simulink model "CPG_component"  (R2021b)
settings: Solver=VariableStepAuto  StartTime=0.0  StopTime=5  RelTol=1e-3
values from neighbouring files (symbols this model uses):
  A = 2    [param.m]
  alpha = 0.856    [param.m]
  epsilon = 5    [param.m]
  f = 1/T    (= 0.8)    [param.m]
  init_state = rand(1, 8)*2 - 1    [param.m]
  k = 1000    [param.m]
  phi_vec = pi*[0; 0.5; 0; 0.5]    [param.m]
  tau = 0.5    [param.m]
settings Model: Creator=kaiget  LastModifiedBy=kaiget

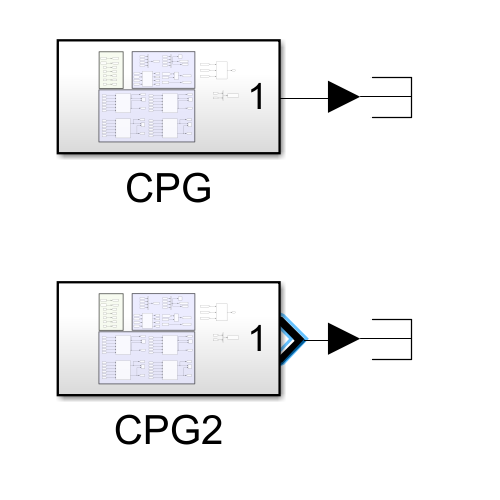
[thumbnail: Simulink's stored preview of the top-level diagram]
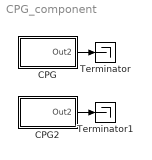
== system CPG_component ==
  CPG : Subsystem
  CPG2 : Subsystem
  Terminator : Terminator
  Terminator1 : Terminator
  wires:
  CPG/1(Out2) -> Terminator/1
  CPG2/1(Out2) -> Terminator1/1

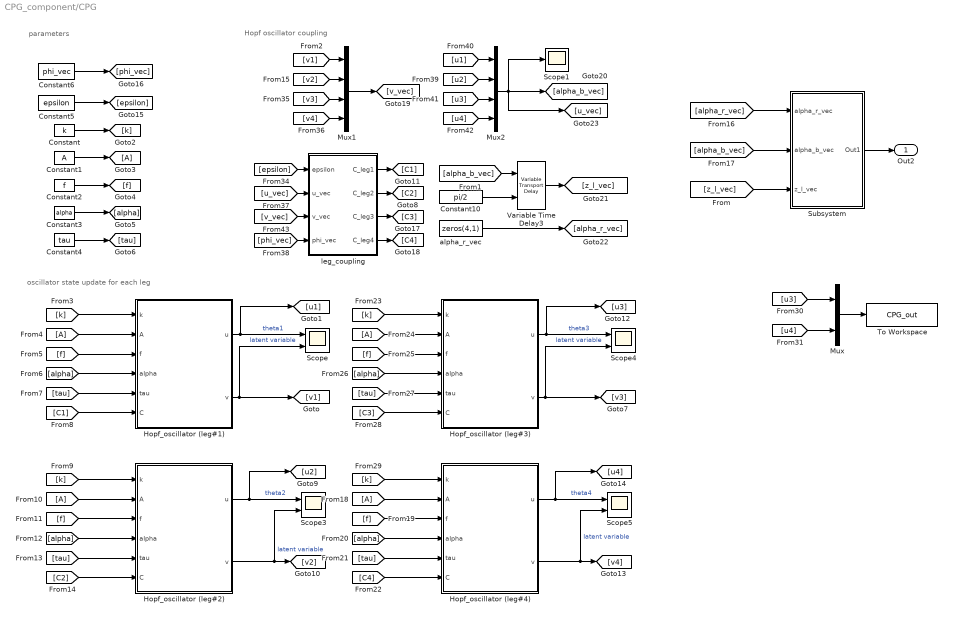
== system CPG_component/CPG ==
  note: oscillator state update for each leg
  note: Hopf oscillator coupling
  note: parameters
  Constant : Constant  Value=k
  Constant1 : Constant  Value=A
  Constant10 : Constant  Value=pi/2
  Constant2 : Constant  Value=f
  Constant3 : Constant  Value=alpha
  Constant4 : Constant  Value=tau
  Constant5 : Constant  Value=epsilon
  Constant6 : Constant  Value=phi_vec
  Hopf_oscillator (leg#1) : Subsystem
  Hopf_oscillator (leg#2) : Subsystem
  Hopf_oscillator (leg#3) : Subsystem
  Hopf_oscillator (leg#4) : Subsystem
  Mux : Mux  Inputs=2
  Mux1 : Mux
  Mux2 : Mux
  Scope{,3..5} (4 alike) : Scope  NumInputPorts=2
  Scope1 : Scope
  Subsystem : Subsystem
  To Workspace : ToWorkspace  VariableName=CPG_out  SaveFormat=Timeseries  SampleTime=0.01
  Variable Time Delay3 : VariableTransportDelay  MaximumDelay=10  MaximumPoints=4096  ZeroDelay=on
  alpha_r_vec : Constant  Value=zeros(4,1)
  leg_coupling : MATLAB Function  TreatAsAtomicUnit=on
  Out2 : Outport
  wires:
  [k] -> Hopf_oscillator (leg#4)/1(k)
  [tau] -> Hopf_oscillator (leg#3)/5(tau)
  [u4] -> Mux2/4
  [v2] -> Mux1/2
  Constant3/1 -> [alpha]
  [epsilon] -> leg_coupling/1(epsilon)
  [u3] -> Mux2/3
  [v_vec] -> leg_coupling/3(v_vec)
  [C2] -> Hopf_oscillator (leg#2)/6(C)
  leg_coupling/4(C_leg4) -> [C4]
  [f] -> Hopf_oscillator (leg#3)/3(f)
  Hopf_oscillator (leg#4)/1(u) -> [u4], Scope5/1  "theta4"
  Hopf_oscillator (leg#4)/2(v) -> [v4], Scope5/2  "latent variable"
  [k] -> Hopf_oscillator (leg#3)/1(k)
  leg_coupling/2(C_leg2) -> [C2]
  Constant2/1 -> [f]
  [u1] -> Mux2/1
  Hopf_oscillator (leg#3)/1(u) -> [u3], Scope4/1  "theta3"
  [A] -> Hopf_oscillator (leg#3)/2(A)
  leg_coupling/3(C_leg3) -> [C3]
  [u2] -> Mux2/2
  Hopf_oscillator (leg#1)/2(v) -> [v1], Scope/2  "latent variable"
  [alpha] -> Hopf_oscillator (leg#2)/4(alpha)
  Hopf_oscillator (leg#3)/2(v) -> [v3], Scope4/2  "latent variable"
  Constant4/1 -> [tau]
  [f] -> Hopf_oscillator (leg#2)/3(f)
  [tau] -> Hopf_oscillator (leg#4)/5(tau)
  [u_vec] -> leg_coupling/2(u_vec)
  [alpha] -> Hopf_oscillator (leg#3)/4(alpha)
  Constant1/1 -> [A]
  [A] -> Hopf_oscillator (leg#1)/2(A)
  [A] -> Hopf_oscillator (leg#2)/2(A)
  leg_coupling/1(C_leg1) -> [C1]
  Mux2/1 -> [u_vec], [alpha_b_vec], Scope1/1
  Hopf_oscillator (leg#2)/1(u) -> [u2], Scope3/1  "theta2"
  [v4] -> Mux1/4
  [f] -> Hopf_oscillator (leg#4)/3(f)
  [C4] -> Hopf_oscillator (leg#4)/6(C)
  [C3] -> Hopf_oscillator (leg#3)/6(C)
  [tau] -> Hopf_oscillator (leg#1)/5(tau)
  Constant5/1 -> [epsilon]
  [A] -> Hopf_oscillator (leg#4)/2(A)
  [k] -> Hopf_oscillator (leg#2)/1(k)
  [alpha] -> Hopf_oscillator (leg#4)/4(alpha)
  [v3] -> Mux1/3
  [k] -> Hopf_oscillator (leg#1)/1(k)
  [phi_vec] -> leg_coupling/4(phi_vec)
  [C1] -> Hopf_oscillator (leg#1)/6(C)
  [v1] -> Mux1/1
  Mux1/1 -> [v_vec]
  [tau] -> Hopf_oscillator (leg#2)/5(tau)
  [f] -> Hopf_oscillator (leg#1)/3(f)
  Constant/1 -> [k]
  Hopf_oscillator (leg#2)/2(v) -> [v2], Scope3/2  "latent variable"
  Hopf_oscillator (leg#1)/1(u) -> [u1], Scope/1  "theta1"
  [alpha] -> Hopf_oscillator (leg#1)/4(alpha)
  Constant6/1 -> [phi_vec]
  [alpha_b_vec] -> Variable Time Delay3/1
  Constant10/1 -> Variable Time Delay3/2
  Variable Time Delay3/1 -> [z_l_vec]
  alpha_r_vec/1 -> [alpha_r_vec]
  [alpha_r_vec] -> Subsystem/1(alpha_r_vec)
  [alpha_b_vec] -> Subsystem/2(alpha_b_vec)
  [z_l_vec] -> Subsystem/3(z_l_vec)
  Subsystem/1(Out1) -> Out2/1
  [u3] -> Mux/1
  [u4] -> Mux/2
  Mux/1 -> To Workspace/1

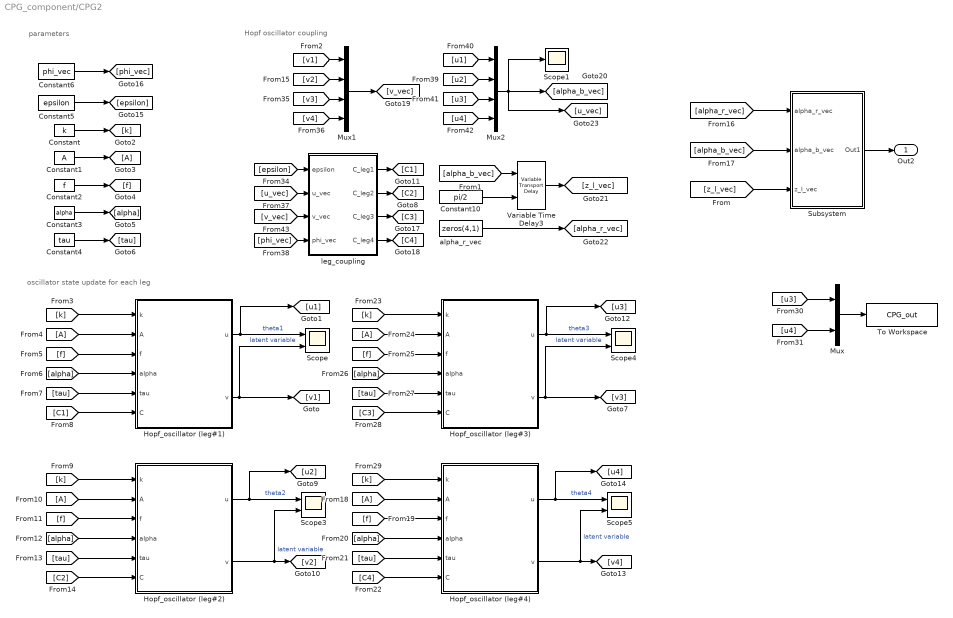
== system CPG_component/CPG2 ==
  note: oscillator state update for each leg
  note: Hopf oscillator coupling
  note: parameters
  Constant : Constant  Value=k
  Constant1 : Constant  Value=A
  Constant10 : Constant  Value=pi/2
  Constant2 : Constant  Value=f
  Constant3 : Constant  Value=alpha
  Constant4 : Constant  Value=tau
  Constant5 : Constant  Value=epsilon
  Constant6 : Constant  Value=phi_vec
  Hopf_oscillator (leg#1) : Subsystem
  Hopf_oscillator (leg#2) : Subsystem
  Hopf_oscillator (leg#3) : Subsystem
  Hopf_oscillator (leg#4) : Subsystem
  Mux : Mux  Inputs=2
  Mux1 : Mux
  Mux2 : Mux
  Scope{,3..5} (4 alike) : Scope  NumInputPorts=2
  Scope1 : Scope
  Subsystem : Subsystem
  To Workspace : ToWorkspace  VariableName=CPG_out  SaveFormat=Timeseries  SampleTime=0.01
  Variable Time Delay3 : VariableTransportDelay  MaximumDelay=10  MaximumPoints=4096  ZeroDelay=on
  alpha_r_vec : Constant  Value=zeros(4,1)
  leg_coupling : MATLAB Function  TreatAsAtomicUnit=on
  Out2 : Outport
  wires:
  [k] -> Hopf_oscillator (leg#4)/1(k)
  [tau] -> Hopf_oscillator (leg#3)/5(tau)
  [u4] -> Mux2/4
  [v2] -> Mux1/2
  Constant3/1 -> [alpha]
  [epsilon] -> leg_coupling/1(epsilon)
  [u3] -> Mux2/3
  [v_vec] -> leg_coupling/3(v_vec)
  [C2] -> Hopf_oscillator (leg#2)/6(C)
  leg_coupling/4(C_leg4) -> [C4]
  [f] -> Hopf_oscillator (leg#3)/3(f)
  Hopf_oscillator (leg#4)/1(u) -> [u4], Scope5/1  "theta4"
  Hopf_oscillator (leg#4)/2(v) -> [v4], Scope5/2  "latent variable"
  [k] -> Hopf_oscillator (leg#3)/1(k)
  leg_coupling/2(C_leg2) -> [C2]
  Constant2/1 -> [f]
  [u1] -> Mux2/1
  Hopf_oscillator (leg#3)/1(u) -> [u3], Scope4/1  "theta3"
  [A] -> Hopf_oscillator (leg#3)/2(A)
  leg_coupling/3(C_leg3) -> [C3]
  [u2] -> Mux2/2
  Hopf_oscillator (leg#1)/2(v) -> [v1], Scope/2  "latent variable"
  [alpha] -> Hopf_oscillator (leg#2)/4(alpha)
  Hopf_oscillator (leg#3)/2(v) -> [v3], Scope4/2  "latent variable"
  Constant4/1 -> [tau]
  [f] -> Hopf_oscillator (leg#2)/3(f)
  [tau] -> Hopf_oscillator (leg#4)/5(tau)
  [u_vec] -> leg_coupling/2(u_vec)
  [alpha] -> Hopf_oscillator (leg#3)/4(alpha)
  Constant1/1 -> [A]
  [A] -> Hopf_oscillator (leg#1)/2(A)
  [A] -> Hopf_oscillator (leg#2)/2(A)
  leg_coupling/1(C_leg1) -> [C1]
  Mux2/1 -> [u_vec], [alpha_b_vec], Scope1/1
  Hopf_oscillator (leg#2)/1(u) -> [u2], Scope3/1  "theta2"
  [v4] -> Mux1/4
  [f] -> Hopf_oscillator (leg#4)/3(f)
  [C4] -> Hopf_oscillator (leg#4)/6(C)
  [C3] -> Hopf_oscillator (leg#3)/6(C)
  [tau] -> Hopf_oscillator (leg#1)/5(tau)
  Constant5/1 -> [epsilon]
  [A] -> Hopf_oscillator (leg#4)/2(A)
  [k] -> Hopf_oscillator (leg#2)/1(k)
  [alpha] -> Hopf_oscillator (leg#4)/4(alpha)
  [v3] -> Mux1/3
  [k] -> Hopf_oscillator (leg#1)/1(k)
  [phi_vec] -> leg_coupling/4(phi_vec)
  [C1] -> Hopf_oscillator (leg#1)/6(C)
  [v1] -> Mux1/1
  Mux1/1 -> [v_vec]
  [tau] -> Hopf_oscillator (leg#2)/5(tau)
  [f] -> Hopf_oscillator (leg#1)/3(f)
  Constant/1 -> [k]
  Hopf_oscillator (leg#2)/2(v) -> [v2], Scope3/2  "latent variable"
  Hopf_oscillator (leg#1)/1(u) -> [u1], Scope/1  "theta1"
  [alpha] -> Hopf_oscillator (leg#1)/4(alpha)
  Constant6/1 -> [phi_vec]
  [alpha_b_vec] -> Variable Time Delay3/1
  Constant10/1 -> Variable Time Delay3/2
  Variable Time Delay3/1 -> [z_l_vec]
  alpha_r_vec/1 -> [alpha_r_vec]
  [alpha_r_vec] -> Subsystem/1(alpha_r_vec)
  [alpha_b_vec] -> Subsystem/2(alpha_b_vec)
  [z_l_vec] -> Subsystem/3(z_l_vec)
  Subsystem/1(Out1) -> Out2/1
  [u3] -> Mux/1
  [u4] -> Mux/2
  Mux/1 -> To Workspace/1

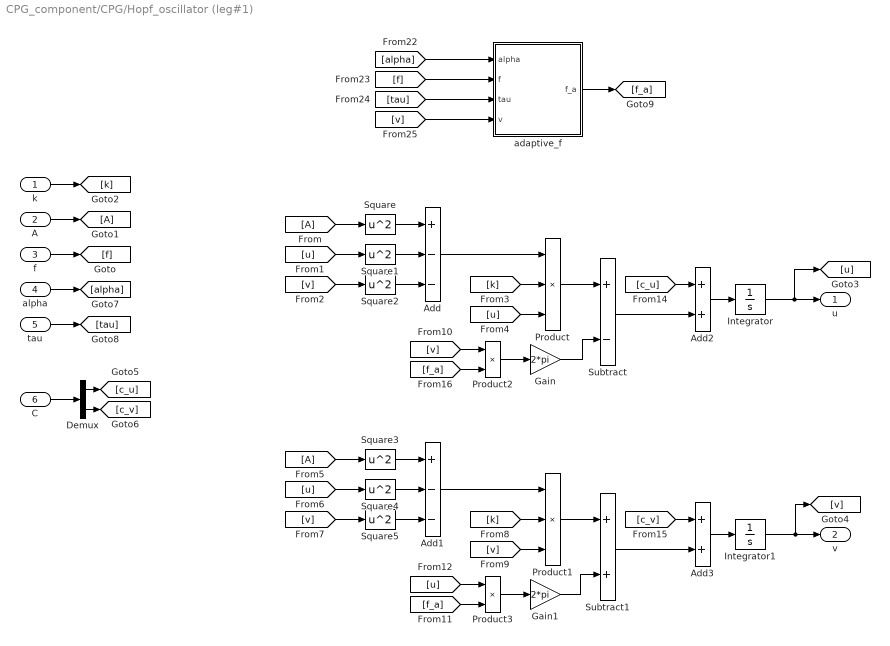
== system CPG_component/CPG/Hopf_oscillator (leg#1) ==
  k : Inport
  A : Inport  Port=2
  f : Inport  Port=3
  alpha : Inport  Port=4
  tau : Inport  Port=5
  C : Inport  Port=6
  Add : Sum  Inputs=+--
  Add1 : Sum  Inputs=+--
  Add2 : Sum
  Add3 : Sum
  Demux : Demux  Outputs=2
  Gain : Gain  Gain=2*pi
  Gain1 : Gain  Gain=2*pi
  Integrator : Integrator  InitialCondition=init_state(1)
  Integrator1 : Integrator  InitialCondition=init_state(2)
  Product : Product  Inputs=3
  Product1 : Product  Inputs=3
  Product2 : Product
  Product3 : Product
  Square{,1..5} (6 alike) : Math  Operator=square  SaturateOnIntegerOverflow=on
  Subtract : Sum  Inputs=+-
  Subtract1 : Sum
  adaptive_f : MATLAB Function  TreatAsAtomicUnit=on
  u : Outport
  v : Outport  Port=2
  wires:
  Integrator/1 -> [u], u/1
  f/1 -> [f]
  A/1 -> [A]
  k/1 -> [k]
  Integrator1/1 -> [v], v/1
  [A] -> Square/1
  [u] -> Square1/1
  [v] -> Square2/1
  Square2/1 -> Add/3
  Square1/1 -> Add/2
  Square/1 -> Add/1
  Add/1 -> Product/1
  [k] -> Product/2
  [u] -> Product/3
  Product/1 -> Subtract/1
  Square3/1 -> Add1/1
  Square4/1 -> Add1/2
  Square5/1 -> Add1/3
  [v] -> Product1/3
  Product1/1 -> Subtract1/1
  [v] -> Square5/1
  [A] -> Square3/1
  [u] -> Square4/1
  Add1/1 -> Product1/1
  [k] -> Product1/2
  [v] -> Product2/1
  [f_a] -> Product2/2
  Product2/1 -> Gain/1
  Gain/1 -> Subtract/2
  [u] -> Product3/1
  Product3/1 -> Gain1/1
  [f_a] -> Product3/2
  Gain1/1 -> Subtract1/2
  Subtract/1 -> Add2/2
  C/1 -> Demux/1
  Demux/1 -> [c_u]
  Demux/2 -> [c_v]
  [c_u] -> Add2/1
  Add2/1 -> Integrator/1
  Subtract1/1 -> Add3/2
  [c_v] -> Add3/1
  Add3/1 -> Integrator1/1
  alpha/1 -> [alpha]
  tau/1 -> [tau]
  [alpha] -> adaptive_f/1(alpha)
  [f] -> adaptive_f/2(f)
  [tau] -> adaptive_f/3(tau)
  [v] -> adaptive_f/4(v)
  adaptive_f/1(f_a) -> [f_a]

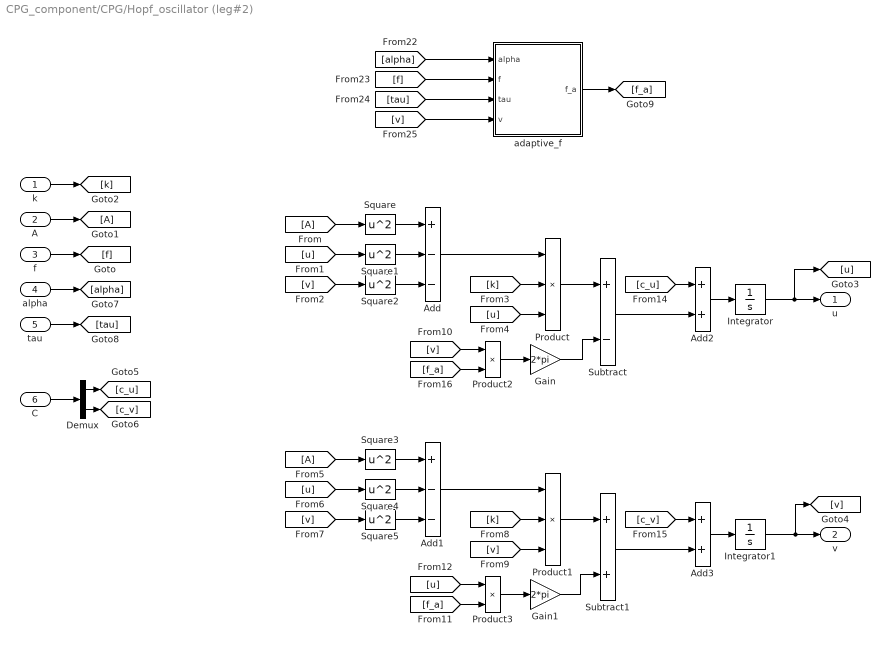
== system CPG_component/CPG/Hopf_oscillator (leg#2) ==
  k : Inport
  A : Inport  Port=2
  f : Inport  Port=3
  alpha : Inport  Port=4
  tau : Inport  Port=5
  C : Inport  Port=6
  Add : Sum  Inputs=+--
  Add1 : Sum  Inputs=+--
  Add2 : Sum
  Add3 : Sum
  Demux : Demux  Outputs=2
  Gain : Gain  Gain=2*pi
  Gain1 : Gain  Gain=2*pi
  Integrator : Integrator  InitialCondition=init_state(3)
  Integrator1 : Integrator  InitialCondition=init_state(4)
  Product : Product  Inputs=3
  Product1 : Product  Inputs=3
  Product2 : Product
  Product3 : Product
  Square{,1..5} (6 alike) : Math  Operator=square  SaturateOnIntegerOverflow=on
  Subtract : Sum  Inputs=+-
  Subtract1 : Sum
  adaptive_f : MATLAB Function  TreatAsAtomicUnit=on
  u : Outport
  v : Outport  Port=2
  wires:
  Integrator/1 -> [u], u/1
  f/1 -> [f]
  A/1 -> [A]
  k/1 -> [k]
  Integrator1/1 -> [v], v/1
  [A] -> Square/1
  [u] -> Square1/1
  [v] -> Square2/1
  Square2/1 -> Add/3
  Square1/1 -> Add/2
  Square/1 -> Add/1
  Add/1 -> Product/1
  [k] -> Product/2
  [u] -> Product/3
  Product/1 -> Subtract/1
  Square3/1 -> Add1/1
  Square4/1 -> Add1/2
  Square5/1 -> Add1/3
  [v] -> Product1/3
  Product1/1 -> Subtract1/1
  [v] -> Square5/1
  [A] -> Square3/1
  [u] -> Square4/1
  Add1/1 -> Product1/1
  [k] -> Product1/2
  [v] -> Product2/1
  [f_a] -> Product2/2
  Product2/1 -> Gain/1
  Gain/1 -> Subtract/2
  [u] -> Product3/1
  Product3/1 -> Gain1/1
  [f_a] -> Product3/2
  Gain1/1 -> Subtract1/2
  Subtract/1 -> Add2/2
  C/1 -> Demux/1
  Demux/1 -> [c_u]
  Demux/2 -> [c_v]
  [c_u] -> Add2/1
  Add2/1 -> Integrator/1
  Subtract1/1 -> Add3/2
  [c_v] -> Add3/1
  Add3/1 -> Integrator1/1
  alpha/1 -> [alpha]
  tau/1 -> [tau]
  [alpha] -> adaptive_f/1(alpha)
  [f] -> adaptive_f/2(f)
  [tau] -> adaptive_f/3(tau)
  [v] -> adaptive_f/4(v)
  adaptive_f/1(f_a) -> [f_a]

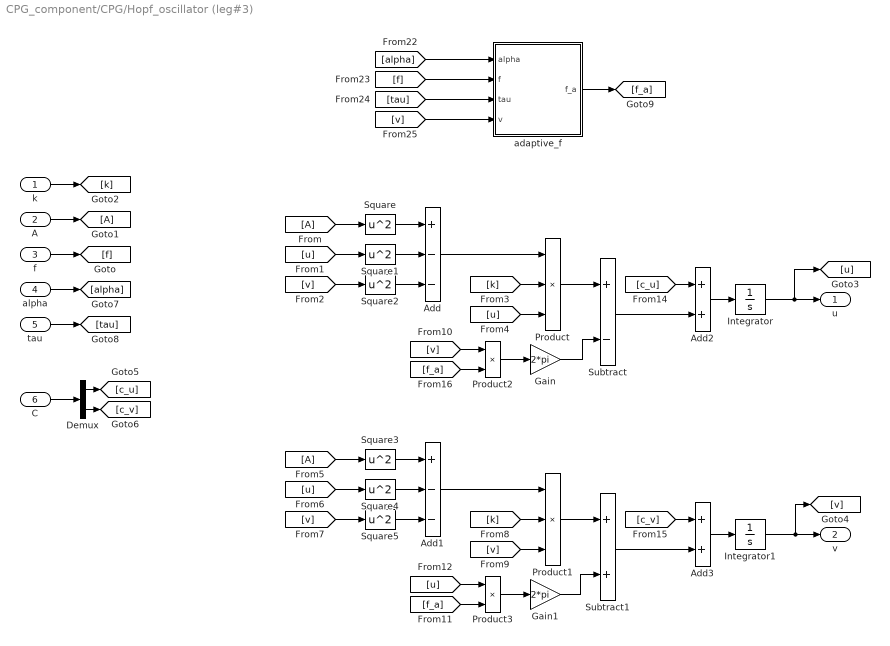
== system CPG_component/CPG/Hopf_oscillator (leg#3) ==
  k : Inport
  A : Inport  Port=2
  f : Inport  Port=3
  alpha : Inport  Port=4
  tau : Inport  Port=5
  C : Inport  Port=6
  Add : Sum  Inputs=+--
  Add1 : Sum  Inputs=+--
  Add2 : Sum
  Add3 : Sum
  Demux : Demux  Outputs=2
  Gain : Gain  Gain=2*pi
  Gain1 : Gain  Gain=2*pi
  Integrator : Integrator  InitialCondition=init_state(5)
  Integrator1 : Integrator  InitialCondition=init_state(6)
  Product : Product  Inputs=3
  Product1 : Product  Inputs=3
  Product2 : Product
  Product3 : Product
  Square{,1..5} (6 alike) : Math  Operator=square  SaturateOnIntegerOverflow=on
  Subtract : Sum  Inputs=+-
  Subtract1 : Sum
  adaptive_f : MATLAB Function  TreatAsAtomicUnit=on
  u : Outport
  v : Outport  Port=2
  wires:
  Integrator/1 -> [u], u/1
  f/1 -> [f]
  A/1 -> [A]
  k/1 -> [k]
  Integrator1/1 -> [v], v/1
  [A] -> Square/1
  [u] -> Square1/1
  [v] -> Square2/1
  Square2/1 -> Add/3
  Square1/1 -> Add/2
  Square/1 -> Add/1
  Add/1 -> Product/1
  [k] -> Product/2
  [u] -> Product/3
  Product/1 -> Subtract/1
  Square3/1 -> Add1/1
  Square4/1 -> Add1/2
  Square5/1 -> Add1/3
  [v] -> Product1/3
  Product1/1 -> Subtract1/1
  [v] -> Square5/1
  [A] -> Square3/1
  [u] -> Square4/1
  Add1/1 -> Product1/1
  [k] -> Product1/2
  [v] -> Product2/1
  [f_a] -> Product2/2
  Product2/1 -> Gain/1
  Gain/1 -> Subtract/2
  [u] -> Product3/1
  Product3/1 -> Gain1/1
  [f_a] -> Product3/2
  Gain1/1 -> Subtract1/2
  Subtract/1 -> Add2/2
  C/1 -> Demux/1
  Demux/1 -> [c_u]
  Demux/2 -> [c_v]
  [c_u] -> Add2/1
  Add2/1 -> Integrator/1
  Subtract1/1 -> Add3/2
  [c_v] -> Add3/1
  Add3/1 -> Integrator1/1
  alpha/1 -> [alpha]
  tau/1 -> [tau]
  [alpha] -> adaptive_f/1(alpha)
  [f] -> adaptive_f/2(f)
  [tau] -> adaptive_f/3(tau)
  [v] -> adaptive_f/4(v)
  adaptive_f/1(f_a) -> [f_a]

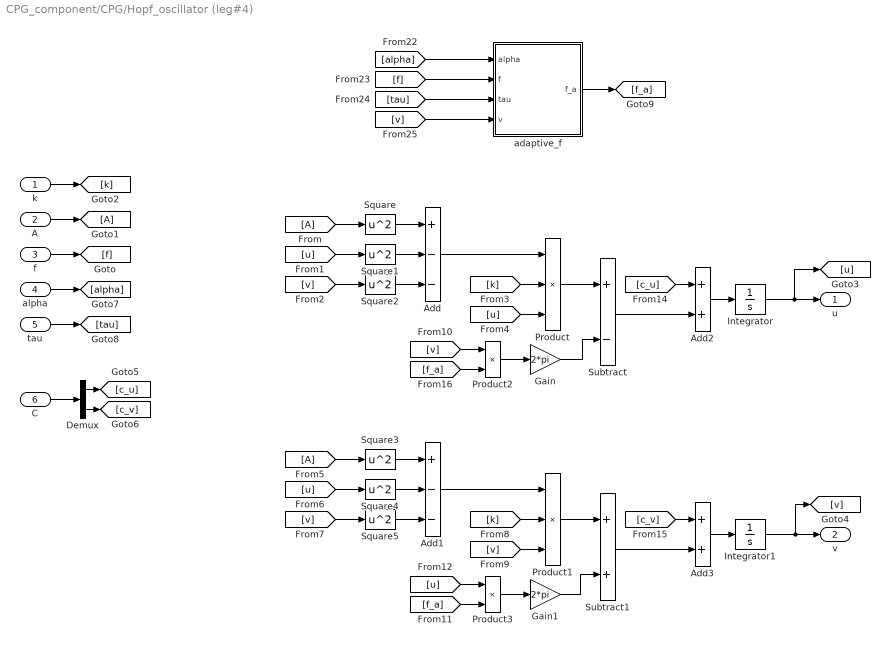
== system CPG_component/CPG/Hopf_oscillator (leg#4) ==
  k : Inport
  A : Inport  Port=2
  f : Inport  Port=3
  alpha : Inport  Port=4
  tau : Inport  Port=5
  C : Inport  Port=6
  Add : Sum  Inputs=+--
  Add1 : Sum  Inputs=+--
  Add2 : Sum
  Add3 : Sum
  Demux : Demux  Outputs=2
  Gain : Gain  Gain=2*pi
  Gain1 : Gain  Gain=2*pi
  Integrator : Integrator  InitialCondition=init_state(7)
  Integrator1 : Integrator  InitialCondition=init_state(8)
  Product : Product  Inputs=3
  Product1 : Product  Inputs=3
  Product2 : Product
  Product3 : Product
  Square{,1..5} (6 alike) : Math  Operator=square  SaturateOnIntegerOverflow=on
  Subtract : Sum  Inputs=+-
  Subtract1 : Sum
  adaptive_f : MATLAB Function  TreatAsAtomicUnit=on
  u : Outport
  v : Outport  Port=2
  wires:
  Integrator/1 -> [u], u/1
  f/1 -> [f]
  A/1 -> [A]
  k/1 -> [k]
  Integrator1/1 -> [v], v/1
  [A] -> Square/1
  [u] -> Square1/1
  [v] -> Square2/1
  Square2/1 -> Add/3
  Square1/1 -> Add/2
  Square/1 -> Add/1
  Add/1 -> Product/1
  [k] -> Product/2
  [u] -> Product/3
  Product/1 -> Subtract/1
  Square3/1 -> Add1/1
  Square4/1 -> Add1/2
  Square5/1 -> Add1/3
  [v] -> Product1/3
  Product1/1 -> Subtract1/1
  [v] -> Square5/1
  [A] -> Square3/1
  [u] -> Square4/1
  Add1/1 -> Product1/1
  [k] -> Product1/2
  [v] -> Product2/1
  [f_a] -> Product2/2
  Product2/1 -> Gain/1
  Gain/1 -> Subtract/2
  [u] -> Product3/1
  Product3/1 -> Gain1/1
  [f_a] -> Product3/2
  Gain1/1 -> Subtract1/2
  Subtract/1 -> Add2/2
  C/1 -> Demux/1
  Demux/1 -> [c_u]
  Demux/2 -> [c_v]
  [c_u] -> Add2/1
  Add2/1 -> Integrator/1
  Subtract1/1 -> Add3/2
  [c_v] -> Add3/1
  Add3/1 -> Integrator1/1
  alpha/1 -> [alpha]
  tau/1 -> [tau]
  [alpha] -> adaptive_f/1(alpha)
  [f] -> adaptive_f/2(f)
  [tau] -> adaptive_f/3(tau)
  [v] -> adaptive_f/4(v)
  adaptive_f/1(f_a) -> [f_a]

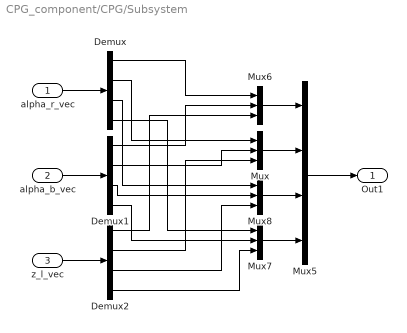
== system CPG_component/CPG/Subsystem ==
  alpha_r_vec : Inport
  alpha_b_vec : Inport  Port=2
  z_l_vec : Inport  Port=3
  Demux : Demux
  Demux1 : Demux
  Demux2 : Demux
  Mux{,6..8} (4 alike) : Mux  Inputs=3
  Mux5 : Mux
  Out1 : Outport
  wires:
  Mux6/1 -> Mux5/1
  Demux1/1 -> Mux6/2
  Demux/3 -> Mux8/1
  Demux2/1 -> Mux6/3
  alpha_b_vec/1 -> Demux1/1
  Demux/1 -> Mux6/1
  Demux2/4 -> Mux7/3
  Demux1/4 -> Mux7/2
  Demux/4 -> Mux7/1
  Mux5/1 -> Out1/1
  Demux2/3 -> Mux8/3
  Demux/2 -> Mux/1
  Mux8/1 -> Mux5/3
  Demux1/3 -> Mux8/2
  Demux1/2 -> Mux/2
  Mux7/1 -> Mux5/4
  Mux/1 -> Mux5/2
  Demux2/2 -> Mux/3
  z_l_vec/1 -> Demux2/1
  alpha_r_vec/1 -> Demux/1

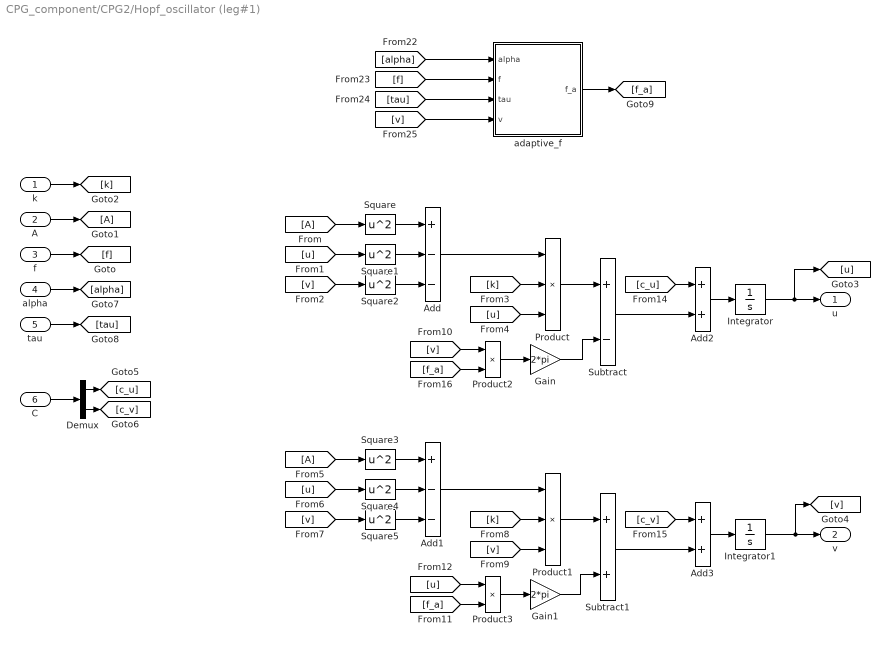
== system CPG_component/CPG2/Hopf_oscillator (leg#1) ==
  k : Inport
  A : Inport  Port=2
  f : Inport  Port=3
  alpha : Inport  Port=4
  tau : Inport  Port=5
  C : Inport  Port=6
  Add : Sum  Inputs=+--
  Add1 : Sum  Inputs=+--
  Add2 : Sum
  Add3 : Sum
  Demux : Demux  Outputs=2
  Gain : Gain  Gain=2*pi
  Gain1 : Gain  Gain=2*pi
  Integrator : Integrator  InitialCondition=init_state(1)
  Integrator1 : Integrator  InitialCondition=init_state(2)
  Product : Product  Inputs=3
  Product1 : Product  Inputs=3
  Product2 : Product
  Product3 : Product
  Square{,1..5} (6 alike) : Math  Operator=square  SaturateOnIntegerOverflow=on
  Subtract : Sum  Inputs=+-
  Subtract1 : Sum
  adaptive_f : MATLAB Function  TreatAsAtomicUnit=on
  u : Outport
  v : Outport  Port=2
  wires:
  Integrator/1 -> [u], u/1
  f/1 -> [f]
  A/1 -> [A]
  k/1 -> [k]
  Integrator1/1 -> [v], v/1
  [A] -> Square/1
  [u] -> Square1/1
  [v] -> Square2/1
  Square2/1 -> Add/3
  Square1/1 -> Add/2
  Square/1 -> Add/1
  Add/1 -> Product/1
  [k] -> Product/2
  [u] -> Product/3
  Product/1 -> Subtract/1
  Square3/1 -> Add1/1
  Square4/1 -> Add1/2
  Square5/1 -> Add1/3
  [v] -> Product1/3
  Product1/1 -> Subtract1/1
  [v] -> Square5/1
  [A] -> Square3/1
  [u] -> Square4/1
  Add1/1 -> Product1/1
  [k] -> Product1/2
  [v] -> Product2/1
  [f_a] -> Product2/2
  Product2/1 -> Gain/1
  Gain/1 -> Subtract/2
  [u] -> Product3/1
  Product3/1 -> Gain1/1
  [f_a] -> Product3/2
  Gain1/1 -> Subtract1/2
  Subtract/1 -> Add2/2
  C/1 -> Demux/1
  Demux/1 -> [c_u]
  Demux/2 -> [c_v]
  [c_u] -> Add2/1
  Add2/1 -> Integrator/1
  Subtract1/1 -> Add3/2
  [c_v] -> Add3/1
  Add3/1 -> Integrator1/1
  alpha/1 -> [alpha]
  tau/1 -> [tau]
  [alpha] -> adaptive_f/1(alpha)
  [f] -> adaptive_f/2(f)
  [tau] -> adaptive_f/3(tau)
  [v] -> adaptive_f/4(v)
  adaptive_f/1(f_a) -> [f_a]

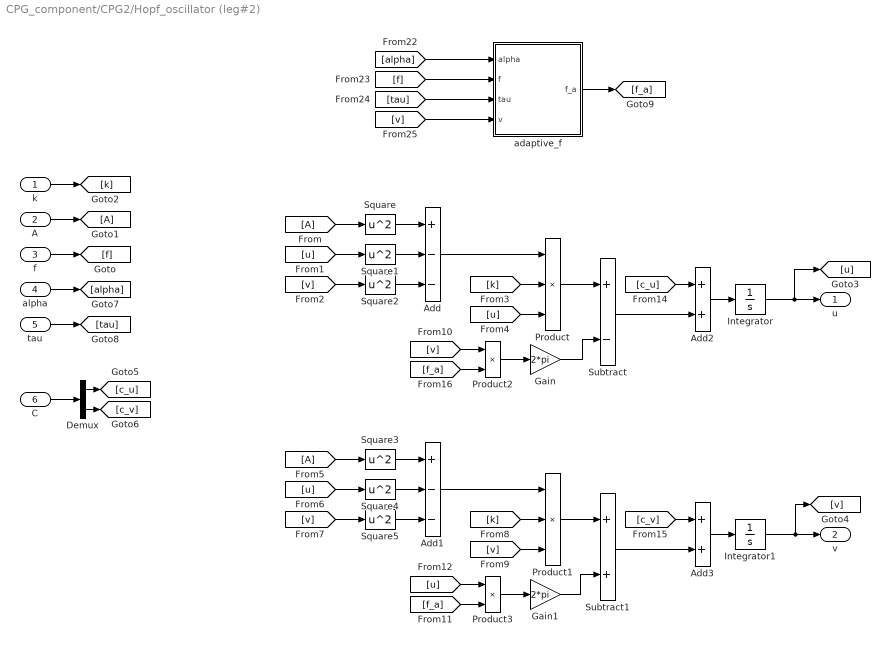
== system CPG_component/CPG2/Hopf_oscillator (leg#2) ==
  k : Inport
  A : Inport  Port=2
  f : Inport  Port=3
  alpha : Inport  Port=4
  tau : Inport  Port=5
  C : Inport  Port=6
  Add : Sum  Inputs=+--
  Add1 : Sum  Inputs=+--
  Add2 : Sum
  Add3 : Sum
  Demux : Demux  Outputs=2
  Gain : Gain  Gain=2*pi
  Gain1 : Gain  Gain=2*pi
  Integrator : Integrator  InitialCondition=init_state(3)
  Integrator1 : Integrator  InitialCondition=init_state(4)
  Product : Product  Inputs=3
  Product1 : Product  Inputs=3
  Product2 : Product
  Product3 : Product
  Square{,1..5} (6 alike) : Math  Operator=square  SaturateOnIntegerOverflow=on
  Subtract : Sum  Inputs=+-
  Subtract1 : Sum
  adaptive_f : MATLAB Function  TreatAsAtomicUnit=on
  u : Outport
  v : Outport  Port=2
  wires:
  Integrator/1 -> [u], u/1
  f/1 -> [f]
  A/1 -> [A]
  k/1 -> [k]
  Integrator1/1 -> [v], v/1
  [A] -> Square/1
  [u] -> Square1/1
  [v] -> Square2/1
  Square2/1 -> Add/3
  Square1/1 -> Add/2
  Square/1 -> Add/1
  Add/1 -> Product/1
  [k] -> Product/2
  [u] -> Product/3
  Product/1 -> Subtract/1
  Square3/1 -> Add1/1
  Square4/1 -> Add1/2
  Square5/1 -> Add1/3
  [v] -> Product1/3
  Product1/1 -> Subtract1/1
  [v] -> Square5/1
  [A] -> Square3/1
  [u] -> Square4/1
  Add1/1 -> Product1/1
  [k] -> Product1/2
  [v] -> Product2/1
  [f_a] -> Product2/2
  Product2/1 -> Gain/1
  Gain/1 -> Subtract/2
  [u] -> Product3/1
  Product3/1 -> Gain1/1
  [f_a] -> Product3/2
  Gain1/1 -> Subtract1/2
  Subtract/1 -> Add2/2
  C/1 -> Demux/1
  Demux/1 -> [c_u]
  Demux/2 -> [c_v]
  [c_u] -> Add2/1
  Add2/1 -> Integrator/1
  Subtract1/1 -> Add3/2
  [c_v] -> Add3/1
  Add3/1 -> Integrator1/1
  alpha/1 -> [alpha]
  tau/1 -> [tau]
  [alpha] -> adaptive_f/1(alpha)
  [f] -> adaptive_f/2(f)
  [tau] -> adaptive_f/3(tau)
  [v] -> adaptive_f/4(v)
  adaptive_f/1(f_a) -> [f_a]

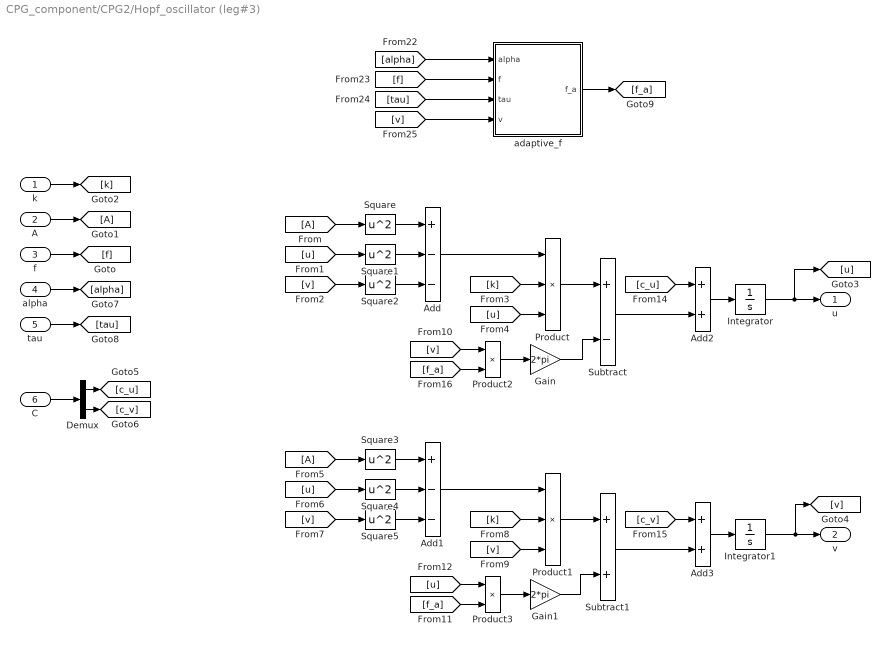
== system CPG_component/CPG2/Hopf_oscillator (leg#3) ==
  k : Inport
  A : Inport  Port=2
  f : Inport  Port=3
  alpha : Inport  Port=4
  tau : Inport  Port=5
  C : Inport  Port=6
  Add : Sum  Inputs=+--
  Add1 : Sum  Inputs=+--
  Add2 : Sum
  Add3 : Sum
  Demux : Demux  Outputs=2
  Gain : Gain  Gain=2*pi
  Gain1 : Gain  Gain=2*pi
  Integrator : Integrator  InitialCondition=init_state(5)
  Integrator1 : Integrator  InitialCondition=init_state(6)
  Product : Product  Inputs=3
  Product1 : Product  Inputs=3
  Product2 : Product
  Product3 : Product
  Square{,1..5} (6 alike) : Math  Operator=square  SaturateOnIntegerOverflow=on
  Subtract : Sum  Inputs=+-
  Subtract1 : Sum
  adaptive_f : MATLAB Function  TreatAsAtomicUnit=on
  u : Outport
  v : Outport  Port=2
  wires:
  Integrator/1 -> [u], u/1
  f/1 -> [f]
  A/1 -> [A]
  k/1 -> [k]
  Integrator1/1 -> [v], v/1
  [A] -> Square/1
  [u] -> Square1/1
  [v] -> Square2/1
  Square2/1 -> Add/3
  Square1/1 -> Add/2
  Square/1 -> Add/1
  Add/1 -> Product/1
  [k] -> Product/2
  [u] -> Product/3
  Product/1 -> Subtract/1
  Square3/1 -> Add1/1
  Square4/1 -> Add1/2
  Square5/1 -> Add1/3
  [v] -> Product1/3
  Product1/1 -> Subtract1/1
  [v] -> Square5/1
  [A] -> Square3/1
  [u] -> Square4/1
  Add1/1 -> Product1/1
  [k] -> Product1/2
  [v] -> Product2/1
  [f_a] -> Product2/2
  Product2/1 -> Gain/1
  Gain/1 -> Subtract/2
  [u] -> Product3/1
  Product3/1 -> Gain1/1
  [f_a] -> Product3/2
  Gain1/1 -> Subtract1/2
  Subtract/1 -> Add2/2
  C/1 -> Demux/1
  Demux/1 -> [c_u]
  Demux/2 -> [c_v]
  [c_u] -> Add2/1
  Add2/1 -> Integrator/1
  Subtract1/1 -> Add3/2
  [c_v] -> Add3/1
  Add3/1 -> Integrator1/1
  alpha/1 -> [alpha]
  tau/1 -> [tau]
  [alpha] -> adaptive_f/1(alpha)
  [f] -> adaptive_f/2(f)
  [tau] -> adaptive_f/3(tau)
  [v] -> adaptive_f/4(v)
  adaptive_f/1(f_a) -> [f_a]

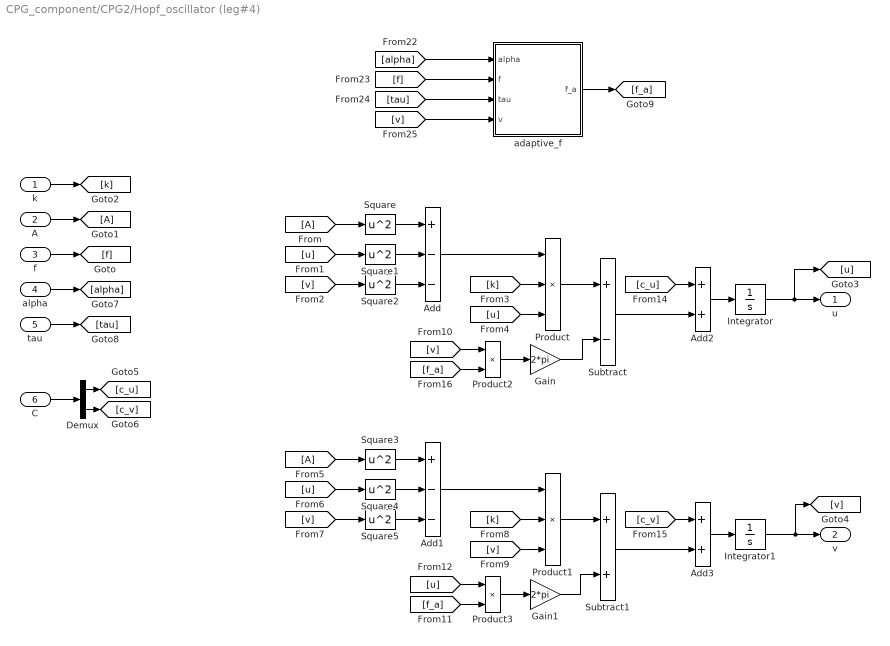
== system CPG_component/CPG2/Hopf_oscillator (leg#4) ==
  k : Inport
  A : Inport  Port=2
  f : Inport  Port=3
  alpha : Inport  Port=4
  tau : Inport  Port=5
  C : Inport  Port=6
  Add : Sum  Inputs=+--
  Add1 : Sum  Inputs=+--
  Add2 : Sum
  Add3 : Sum
  Demux : Demux  Outputs=2
  Gain : Gain  Gain=2*pi
  Gain1 : Gain  Gain=2*pi
  Integrator : Integrator  InitialCondition=init_state(7)
  Integrator1 : Integrator  InitialCondition=init_state(8)
  Product : Product  Inputs=3
  Product1 : Product  Inputs=3
  Product2 : Product
  Product3 : Product
  Square{,1..5} (6 alike) : Math  Operator=square  SaturateOnIntegerOverflow=on
  Subtract : Sum  Inputs=+-
  Subtract1 : Sum
  adaptive_f : MATLAB Function  TreatAsAtomicUnit=on
  u : Outport
  v : Outport  Port=2
  wires:
  Integrator/1 -> [u], u/1
  f/1 -> [f]
  A/1 -> [A]
  k/1 -> [k]
  Integrator1/1 -> [v], v/1
  [A] -> Square/1
  [u] -> Square1/1
  [v] -> Square2/1
  Square2/1 -> Add/3
  Square1/1 -> Add/2
  Square/1 -> Add/1
  Add/1 -> Product/1
  [k] -> Product/2
  [u] -> Product/3
  Product/1 -> Subtract/1
  Square3/1 -> Add1/1
  Square4/1 -> Add1/2
  Square5/1 -> Add1/3
  [v] -> Product1/3
  Product1/1 -> Subtract1/1
  [v] -> Square5/1
  [A] -> Square3/1
  [u] -> Square4/1
  Add1/1 -> Product1/1
  [k] -> Product1/2
  [v] -> Product2/1
  [f_a] -> Product2/2
  Product2/1 -> Gain/1
  Gain/1 -> Subtract/2
  [u] -> Product3/1
  Product3/1 -> Gain1/1
  [f_a] -> Product3/2
  Gain1/1 -> Subtract1/2
  Subtract/1 -> Add2/2
  C/1 -> Demux/1
  Demux/1 -> [c_u]
  Demux/2 -> [c_v]
  [c_u] -> Add2/1
  Add2/1 -> Integrator/1
  Subtract1/1 -> Add3/2
  [c_v] -> Add3/1
  Add3/1 -> Integrator1/1
  alpha/1 -> [alpha]
  tau/1 -> [tau]
  [alpha] -> adaptive_f/1(alpha)
  [f] -> adaptive_f/2(f)
  [tau] -> adaptive_f/3(tau)
  [v] -> adaptive_f/4(v)
  adaptive_f/1(f_a) -> [f_a]

== system CPG_component/CPG2/Subsystem ==
  alpha_r_vec : Inport
  alpha_b_vec : Inport  Port=2
  z_l_vec : Inport  Port=3
  Demux : Demux
  Demux1 : Demux
  Demux2 : Demux
  Mux{,6..8} (4 alike) : Mux  Inputs=3
  Mux5 : Mux
  Out1 : Outport
  wires:
  Mux6/1 -> Mux5/1
  Demux1/1 -> Mux6/2
  Demux/3 -> Mux8/1
  Demux2/1 -> Mux6/3
  alpha_b_vec/1 -> Demux1/1
  Demux/1 -> Mux6/1
  Demux2/4 -> Mux7/3
  Demux1/4 -> Mux7/2
  Demux/4 -> Mux7/1
  Mux5/1 -> Out1/1
  Demux2/3 -> Mux8/3
  Demux/2 -> Mux/1
  Mux8/1 -> Mux5/3
  Demux1/3 -> Mux8/2
  Demux1/2 -> Mux/2
  Mux7/1 -> Mux5/4
  Mux/1 -> Mux5/2
  Demux2/2 -> Mux/3
  z_l_vec/1 -> Demux2/1
  alpha_r_vec/1 -> Demux/1

== matlab function CPG_component/CPG/leg_coupling ==
  data: epsilon input; u_vec input; C_leg1 output size=2; v_vec input; phi_vec input; C_leg2 output size=2; C_leg3 output size=2; C_leg4 output size=2
% epsilon: 1X1
% u_vec: 4X1
% v_vec: 4X1
% phi_vec: 4X1
% C_leg1-4 : 2X1
function [C_leg1, C_leg2, C_leg3, C_leg4] = fcn(epsilon, u_vec, v_vec, phi_vec)
    C1 = 0;
    % first leg
    C21 = epsilon*(-u_vec(4)*sin(phi_vec(4)) + v_vec(4)*cos(phi_vec(4)) - ...
                   -u_vec(1)*sin(phi_vec(1)) + v_vec(2)*cos(phi_vec(1)));
    C22 = epsilon*(-u_vec(1)*sin(phi_vec(1)) + v_vec(1)*cos(phi_vec(1)) - ...
                   -u_vec(2)*sin(phi_vec(2)) + v_vec(3)*cos(phi_vec(2)));
    C23 = epsilon*(-u_vec(2)*sin(phi_vec(2)) + v_vec(2)*cos(phi_vec(2)) - ...
                   -u_vec(3)*sin(phi_vec(3)) + v_vec(4)*cos(phi_vec(3)));
    C24 = epsilon*(-u_vec(3)*sin(phi_vec(3)) + v_vec(3)*cos(phi_vec(3)) - ...
                   -u_vec(4)*sin(phi_vec(4)) + v_vec(1)*cos(phi_vec(4)));
    
    C_leg1 = [C1; C21];
    C_leg2 = [C1; C22];
    C_leg3 = [C1; C23];
    C_leg4 = [C1; C24];

== matlab function CPG_component/CPG2/Hopf_oscillator (leg#1)/adaptive_f ==
  data: alpha input; f_a output; f input; tau input; v input
 % calculate the adaptive frequency f through (4) in 
 % 'Design and Locomotion Control of a Biomimetic Underwater Vehicle ... '
function f_a = adaptive_f(alpha, f, tau, v)
    f1 = f/2/alpha;
    f2 = (2*alpha - 1)*f/(2*alpha*(1 - alpha)*(1 + exp(-tau*v)));
    f_a = f1 + f2;

== matlab function CPG_component/CPG2/Hopf_oscillator (leg#2)/adaptive_f ==
  data: alpha input; f_a output; f input; tau input; v input
 % calculate the adaptive frequency f through (4) in 
 % 'Design and Locomotion Control of a Biomimetic Underwater Vehicle ... '
function f_a = adaptive_f(alpha, f, tau, v)
    f1 = f/2/alpha;
    f2 = (2*alpha - 1)*f/(2*alpha*(1 - alpha)*(1 + exp(-tau*v)));
    f_a = f1 + f2;

== matlab function CPG_component/CPG2/Hopf_oscillator (leg#3)/adaptive_f ==
  data: alpha input; f_a output; f input; tau input; v input
 % calculate the adaptive frequency f through (4) in 
 % 'Design and Locomotion Control of a Biomimetic Underwater Vehicle ... '
function f_a = adaptive_f(alpha, f, tau, v)
    f1 = f/2/alpha;
    f2 = (2*alpha - 1)*f/(2*alpha*(1 - alpha)*(1 + exp(-tau*v)));
    f_a = f1 + f2;

== matlab function CPG_component/CPG2/Hopf_oscillator (leg#4)/adaptive_f ==
  data: alpha input; f_a output; f input; tau input; v input
 % calculate the adaptive frequency f through (4) in 
 % 'Design and Locomotion Control of a Biomimetic Underwater Vehicle ... '
function f_a = adaptive_f(alpha, f, tau, v)
    f1 = f/2/alpha;
    f2 = (2*alpha - 1)*f/(2*alpha*(1 - alpha)*(1 + exp(-tau*v)));
    f_a = f1 + f2;

== matlab function CPG_component/CPG2/leg_coupling ==
  data: epsilon input; u_vec input; C_leg1 output size=2; v_vec input; phi_vec input; C_leg2 output size=2; C_leg3 output size=2; C_leg4 output size=2
% epsilon: 1X1
% u_vec: 4X1
% v_vec: 4X1
% phi_vec: 4X1
% C_leg1-4 : 2X1
function [C_leg1, C_leg2, C_leg3, C_leg4] = fcn(epsilon, u_vec, v_vec, phi_vec)
    C1 = 0;
    % first leg
    C21 = 0;
    C22 = epsilon*(u_vec(1)*sin(phi_vec(2)) + v_vec(1)*cos(phi_vec(2)));
    C23 = epsilon*(u_vec(1)*sin(phi_vec(3)) + v_vec(1)*cos(phi_vec(3)));
    C24 = epsilon*(u_vec(1)*sin(phi_vec(4)) + v_vec(1)*cos(phi_vec(4)));
    
    C_leg1 = [C1; C21];
    C_leg2 = [C1; C22];
    C_leg3 = [C1; C23];
    C_leg4 = [C1; C24];

== matlab function CPG_component/CPG/Hopf_oscillator (leg#1)/adaptive_f ==
  data: alpha input; f_a output; f input; tau input; v input
 % calculate the adaptive frequency f through (4) in 
 % 'Design and Locomotion Control of a Biomimetic Underwater Vehicle ... '
function f_a = adaptive_f(alpha, f, tau, v)
    f1 = f/2/alpha;
    f2 = (2*alpha - 1)*f/(2*alpha*(1 - alpha)*(1 + exp(-tau*v)));
    f_a = f1 + f2;

== matlab function CPG_component/CPG/Hopf_oscillator (leg#2)/adaptive_f ==
  data: alpha input; f_a output; f input; tau input; v input
 % calculate the adaptive frequency f through (4) in 
 % 'Design and Locomotion Control of a Biomimetic Underwater Vehicle ... '
function f_a = adaptive_f(alpha, f, tau, v)
    f1 = f/2/alpha;
    f2 = (2*alpha - 1)*f/(2*alpha*(1 - alpha)*(1 + exp(-tau*v)));
    f_a = f1 + f2;

== matlab function CPG_component/CPG/Hopf_oscillator (leg#3)/adaptive_f ==
  data: alpha input; f_a output; f input; tau input; v input
 % calculate the adaptive frequency f through (4) in 
 % 'Design and Locomotion Control of a Biomimetic Underwater Vehicle ... '
function f_a = adaptive_f(alpha, f, tau, v)
    f1 = f/2/alpha;
    f2 = (2*alpha - 1)*f/(2*alpha*(1 - alpha)*(1 + exp(-tau*v)));
    f_a = f1 + f2;

== matlab function CPG_component/CPG/Hopf_oscillator (leg#4)/adaptive_f ==
  data: alpha input; f_a output; f input; tau input; v input
 % calculate the adaptive frequency f through (4) in 
 % 'Design and Locomotion Control of a Biomimetic Underwater Vehicle ... '
function f_a = adaptive_f(alpha, f, tau, v)
    f1 = f/2/alpha;
    f2 = (2*alpha - 1)*f/(2*alpha*(1 - alpha)*(1 + exp(-tau*v)));
    f_a = f1 + f2;
